simulink library "utility_service_lib"  (Simulink 8.1)
settings: Solver=ode45  StartTime=0.0  StopTime=10.0  RelTol=1e-3
values from neighbouring files (symbols this model uses):
  Ts = 100E-6    (= 0.0001)    [BANSHEE_init.m]    (also in Ghost_init.m)
undefined symbols (not defined in the file or in its folder): Left, type, V
libraries: cables_lib x9, breaker_lib x4, transformer_lib x3, rtlab x2, fault_lib x1, ssn_lib x1, controllable_grid_lib x1
settings Model: Creator=RE25624  LastModifiedBy=hptb1

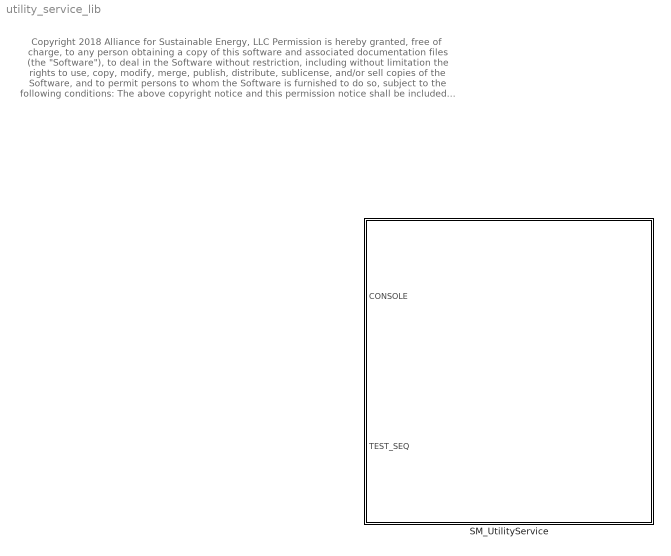
== system utility_service_lib ==
  note: Copyright 2018 Alliance for Sustainable Energy, LLC
      |
      | Permission is hereby granted, free of charge, to any person obtaining a copy of this software
      | and associated documentation files (the "Software"), to deal in the Software without restriction,
      | including without limitation the rights to use, copy, modify, merge, publish, distribute, sublicense,
      | and/or sell copies of the Software, and to permit persons to whom the Software is furnished to do so,
      | subject to the following conditions:
      |
      | The above copyright notice and this permission notice shall be included in all copies or substantial portions of the Software.
      |
      | THE SOFTWARE IS PROVIDED "AS IS", WITHOUT WARRANTY OF ANY KIND, EXPRESS OR IMPLIED, INCLUDING
      | BUT NOT LIMITED TO THE WARRANTIES OF MERCHANTABILITY, FITNESS FOR A PARTICULAR PURPOSE AND
      | NONINFRINGEMENT. IN NO EVENT SHALL THE AUTHORS, THE COPYRIGHT HOLDERS, THE UNITED STATES,
      | THE UNITED STATES DEPARTMENT OF ENERGY, OR ANY OF THEIR EMPLOYEES BE LIABLE FOR ANY CLAIM,
      | DAMAGES OR OTHER LIABILITY, WHETHER IN AN ACTION OF CONTRACT, TORT OR OTHERWISE, ARISING FROM,
      | OUT OF OR IN CONNECTION WITH THE SOFTWARE OR THE USE OR OTHER DEALINGS IN THE SOFTWARE.
  SM_UtilityService : Subsystem

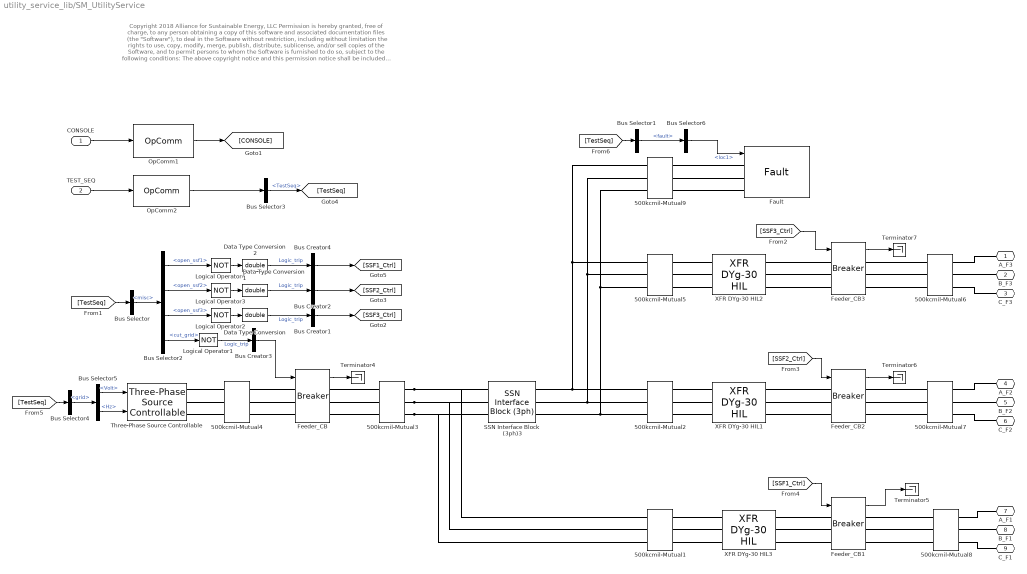
== system utility_service_lib/SM_UtilityService ==
  note: Copyright 2018 Alliance for Sustainable Energy, LLC
      |
      | Permission is hereby granted, free of charge, to any person obtaining a copy of this software
      | and associated documentation files (the "Software"), to deal in the Software without restriction,
      | including without limitation the rights to use, copy, modify, merge, publish, distribute, sublicense,
      | and/or sell copies of the Software, and to permit persons to whom the Software is furnished to do so,
      | subject to the following conditions:
      |
      | The above copyright notice and this permission notice shall be included in all copies or substantial portions of the Software.
      |
      | THE SOFTWARE IS PROVIDED "AS IS", WITHOUT WARRANTY OF ANY KIND, EXPRESS OR IMPLIED, INCLUDING
      | BUT NOT LIMITED TO THE WARRANTIES OF MERCHANTABILITY, FITNESS FOR A PARTICULAR PURPOSE AND
      | NONINFRINGEMENT. IN NO EVENT SHALL THE AUTHORS, THE COPYRIGHT HOLDERS, THE UNITED STATES,
      | THE UNITED STATES DEPARTMENT OF ENERGY, OR ANY OF THEIR EMPLOYEES BE LIABLE FOR ANY CLAIM,
      | DAMAGES OR OTHER LIABILITY, WHETHER IN AN ACTION OF CONTRACT, TORT OR OTHERWISE, ARISING FROM,
      | OUT OF OR IN CONNECTION WITH THE SOFTWARE OR THE USE OR OTHER DEALINGS IN THE SOFTWARE.
  CONSOLE : Inport
  TEST_SEQ : Inport  Port=2
  500kcmil-Mutual{1..2,5,9} (4 alike) : cables_lib/500kcmil-Mutual  length=200  par_sets=1  ratio=3
  500kcmil-Mutual{3..4,6..8} (5 alike) : cables_lib/500kcmil-Mutual  length=50  par_sets=1  ratio=3
  Bus Creator{1..4} (4 alike) : BusCreator  Inputs=1
  Bus Selector : BusSelector  OutputSignals=misc
  Bus Selector1 : BusSelector  OutputSignals=fault
  Bus Selector2 : BusSelector  OutputSignals=open_ssf1,open_ssf2,open_ssf3,cut_grid
  Bus Selector3 : BusSelector  OutputSignals=TestSeq
  Bus Selector4 : BusSelector  OutputSignals=grid
  Bus Selector5 : BusSelector  OutputSignals=Volt,Hz
  Bus Selector6 : BusSelector  OutputSignals=loc1
  Data Type Conversion : DataTypeConversion  OutDataTypeStr=double
  Data Type Conversion1 : DataTypeConversion  OutDataTypeStr=double
  Data Type Conversion2 : DataTypeConversion  OutDataTypeStr=double
  Fault : fault_lib/Fault  FaultResistance=0.1  GroundResistance=1.73  SnubberResistance=1E6
  Feeder_CB{,1..3} (4 alike) : breaker_lib/Breaker  Ts=Ts  mech_delay=cb_mech_delay
  Logical Operator{1..4} (4 alike) : Logic  Operator=NOT  AllPortsSameDT=off  OutDataTypeStr=boolean
  OpComm1 : rtlab/OpComm  nbport=1  groupe_acq=1  subsys_rate=0  st=0  Synchronization=on  Interpolation=on  Threshold=1.0  Missed_Data=off  Sim_Time=off  Samples=off  dynSigOut=off  from_console=1  warning_done=off  writeOpCommFile=off  Offset=off
  OpComm2 : rtlab/OpComm  nbport=1  groupe_acq=1  subsys_rate=0  st=0  Synchronization=on  Interpolation=on  Threshold=1.0  Missed_Data=off  Sim_Time=off  Samples=off  dynSigOut=off  from_console=0  warning_done=off  writeOpCommFile=off  Offset=off
  SSN Interface Block (3ph)3 : ssn_lib/SSN Interface Block (3ph)  nb_phase=3  nb_port=2  p1_type=V-type(Left)  p2_type=V-type (Right)  p3_type=V-type(Left)  p4_type=V-type(Left)  p5_type=V-type(Left)  p6_type=V-type(Left)  p7_type=V-type(Left)  p8_type=V-type(Left)  p9_type=V-type(Left)  p10_type=V-type(Left)  p11_type=V-type(Left)  p12_type=V-type(Left)  p13_type=V-type(Left)  p14_type=V-type(Left)  p15_type=V-type(Left)  p16_type=V-type(Left)  I_port_shunt_resistance=1e9
  Terminator{4..7} (4 alike) : Terminator
  Three-Phase Source Controllable : controllable_grid_lib/Three-Phase Source Controllable  Ts=Ts  Rg=0.8  Lg=16.58e-3  mask{Ts=Ts}
  XFR DYg-30 HIL1 : transformer_lib/XFR DYg-30 HIL  Rating=50000  Vp=115000  Vs=13800  Z=6  XR=30
  XFR DYg-30 HIL2 : transformer_lib/XFR DYg-30 HIL  Rating=50000  Vp=115000  Vs=13800  Z=6  XR=30
  XFR DYg-30 HIL3 : transformer_lib/XFR DYg-30 HIL  Rating=50000  Vp=115000  Vs=13800  Z=6  XR=30
  A_F3 : PMIOPort  Port=1  Side=Right
  B_F3 : PMIOPort  Port=2  Side=Right
  C_F3 : PMIOPort  Port=3  Side=Right
  A_F2 : PMIOPort  Port=4  Side=Right
  B_F2 : PMIOPort  Port=5  Side=Right
  C_F2 : PMIOPort  Port=6  Side=Right
  A_F1 : PMIOPort  Port=7  Side=Right
  B_F1 : PMIOPort  Port=8  Side=Right
  C_F1 : PMIOPort  Port=9  Side=Right
  wires:
  Bus Selector6/1 -> Fault/1  "<loc1>"
  Bus Selector1/1 -> Bus Selector6/1  "<fault>"
  [TestSeq] -> Bus Selector1/1
  Bus Selector5/1 -> Three-Phase Source Controllable/1  "<Volt>"
  Bus Selector5/2 -> Three-Phase Source Controllable/2  "<Hz>"
  Bus Selector4/1 -> Bus Selector5/1  "<grid>"
  [TestSeq] -> Bus Selector4/1
  [SSF1_Ctrl] -> Feeder_CB1/1
  [SSF2_Ctrl] -> Feeder_CB2/1
  [SSF3_Ctrl] -> Feeder_CB3/1
  Data Type Conversion2/1 -> Bus Creator4/1  "Logic_trip"
  Bus Creator4/1 -> [SSF1_Ctrl]
  Logical Operator4/1 -> Data Type Conversion2/1
  Bus Selector2/1 -> Logical Operator4/1  "<open_ssf1>"
  Data Type Conversion1/1 -> Bus Creator2/1  "Logic_trip"
  Bus Creator2/1 -> [SSF2_Ctrl]
  Logical Operator3/1 -> Data Type Conversion1/1
  Bus Selector2/2 -> Logical Operator3/1  "<open_ssf2>"
  OpComm2/1 -> Bus Selector3/1
  Bus Selector3/1 -> [TestSeq]  "<TestSeq>"
  Data Type Conversion/1 -> Bus Creator1/1  "Logic_trip"
  Bus Creator1/1 -> [SSF3_Ctrl]
  Logical Operator2/1 -> Data Type Conversion/1
  Bus Selector2/3 -> Logical Operator2/1  "<open_ssf3>"
  Bus Selector2/4 -> Logical Operator1/1  "<cut_grid>"
  Bus Selector/1 -> Bus Selector2/1  "<misc>"
  Bus Creator3/1 -> Feeder_CB/1
  Logical Operator1/1 -> Bus Creator3/1  "Logic_trip"
  [TestSeq] -> Bus Selector/1
  TEST_SEQ/1 -> OpComm2/1
  Feeder_CB3/1 -> Terminator7/1
  Feeder_CB2/1 -> Terminator6/1
  Feeder_CB1/1 -> Terminator5/1
  Feeder_CB/1 -> Terminator4/1
  OpComm1/1 -> [CONSOLE]
  CONSOLE/1 -> OpComm1/1
  connections:
  500kcmil-Mutual9/RConn1 -- Fault/LConn1
  500kcmil-Mutual9/RConn3 -- Fault/LConn3
  500kcmil-Mutual9/RConn2 -- Fault/LConn2
  C_F3/RConn1 -- 500kcmil-Mutual6/RConn3
  A_F3/RConn1 -- 500kcmil-Mutual6/RConn1
  B_F3/RConn1 -- 500kcmil-Mutual6/RConn2
  C_F2/RConn1 -- 500kcmil-Mutual7/RConn3
  A_F2/RConn1 -- 500kcmil-Mutual7/RConn1
  B_F2/RConn1 -- 500kcmil-Mutual7/RConn2
  A_F1/RConn1 -- 500kcmil-Mutual8/RConn1
  C_F1/RConn1 -- 500kcmil-Mutual8/RConn3
  B_F1/RConn1 -- 500kcmil-Mutual8/RConn2
  500kcmil-Mutual8/LConn3 -- Feeder_CB1/RConn3
  500kcmil-Mutual8/LConn2 -- Feeder_CB1/RConn2
  500kcmil-Mutual8/LConn1 -- Feeder_CB1/RConn1
  500kcmil-Mutual7/LConn1 -- Feeder_CB2/RConn1
  500kcmil-Mutual7/LConn3 -- Feeder_CB2/RConn3
  500kcmil-Mutual7/LConn2 -- Feeder_CB2/RConn2
  500kcmil-Mutual6/LConn1 -- Feeder_CB3/RConn1
  500kcmil-Mutual6/LConn3 -- Feeder_CB3/RConn3
  500kcmil-Mutual6/LConn2 -- Feeder_CB3/RConn2
  Feeder_CB1/LConn1 -- XFR DYg-30 HIL3/RConn1
  Feeder_CB1/LConn2 -- XFR DYg-30 HIL3/RConn2
  Feeder_CB1/LConn3 -- XFR DYg-30 HIL3/RConn3
  XFR DYg-30 HIL1/RConn1 -- Feeder_CB2/LConn1
  XFR DYg-30 HIL1/RConn2 -- Feeder_CB2/LConn2
  XFR DYg-30 HIL1/RConn3 -- Feeder_CB2/LConn3
  XFR DYg-30 HIL2/RConn3 -- Feeder_CB3/LConn3
  XFR DYg-30 HIL2/RConn2 -- Feeder_CB3/LConn2
  XFR DYg-30 HIL2/RConn1 -- Feeder_CB3/LConn1
  500kcmil-Mutual9/LConn3 -- 500kcmil-Mutual2/LConn3 -- SSN Interface Block (3ph)3/RConn3 -- 500kcmil-Mutual5/LConn3
  500kcmil-Mutual9/LConn2 -- 500kcmil-Mutual2/LConn2 -- SSN Interface Block (3ph)3/RConn2 -- 500kcmil-Mutual5/LConn2
  500kcmil-Mutual9/LConn1 -- 500kcmil-Mutual5/LConn1 -- 500kcmil-Mutual2/LConn1 -- SSN Interface Block (3ph)3/RConn1
  500kcmil-Mutual1/RConn1 -- XFR DYg-30 HIL3/LConn1
  500kcmil-Mutual1/RConn2 -- XFR DYg-30 HIL3/LConn2
  500kcmil-Mutual1/RConn3 -- XFR DYg-30 HIL3/LConn3
  500kcmil-Mutual5/RConn3 -- XFR DYg-30 HIL2/LConn3
  500kcmil-Mutual5/RConn1 -- XFR DYg-30 HIL2/LConn1
  500kcmil-Mutual5/RConn2 -- XFR DYg-30 HIL2/LConn2
  500kcmil-Mutual2/RConn3 -- XFR DYg-30 HIL1/LConn3
  500kcmil-Mutual2/RConn1 -- XFR DYg-30 HIL1/LConn1
  500kcmil-Mutual2/RConn2 -- XFR DYg-30 HIL1/LConn2
  Three-Phase Source Controllable/RConn2 -- 500kcmil-Mutual4/LConn2
  Three-Phase Source Controllable/RConn1 -- 500kcmil-Mutual4/LConn1
  Three-Phase Source Controllable/RConn3 -- 500kcmil-Mutual4/LConn3
  500kcmil-Mutual4/RConn1 -- Feeder_CB/LConn1
  500kcmil-Mutual4/RConn2 -- Feeder_CB/LConn2
  500kcmil-Mutual4/RConn3 -- Feeder_CB/LConn3
  500kcmil-Mutual3/RConn3 -- 500kcmil-Mutual1/LConn3 -- SSN Interface Block (3ph)3/LConn3
  500kcmil-Mutual3/RConn1 -- 500kcmil-Mutual1/LConn1 -- SSN Interface Block (3ph)3/LConn1
  500kcmil-Mutual3/RConn2 -- 500kcmil-Mutual1/LConn2 -- SSN Interface Block (3ph)3/LConn2
  500kcmil-Mutual3/LConn2 -- Feeder_CB/RConn2
  500kcmil-Mutual3/LConn1 -- Feeder_CB/RConn1
  500kcmil-Mutual3/LConn3 -- Feeder_CB/RConn3
